simulink model "SMPMSM"  (R2018a)
settings: Solver=VariableStepAuto  StartTime=0.0  StopTime=1  MaxStep=1e-5  RelTol=1e-3
libraries: powerlib x27, simulink x5, powerlib_meascontrol x2
settings Model: Creator=Ogün Altun  LastModifiedBy=Ogün Altun
settings SolverCC: ZeroCrossAlgorithm=Adaptive
settings DebuggingCC: MaxConsecutiveZCsMsg=none

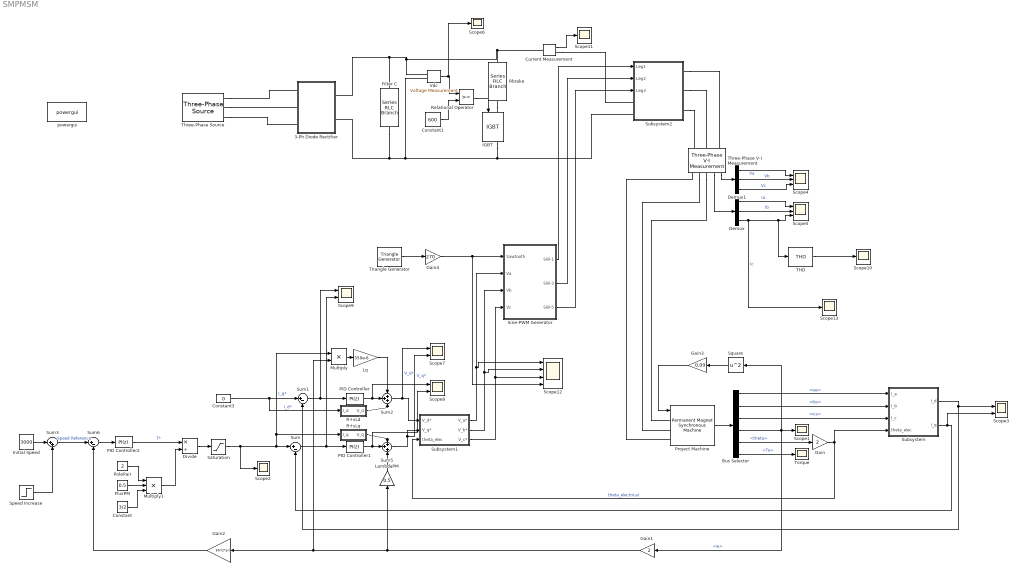
== system SMPMSM ==
  3-Ph Diode Rectifier : Subsystem
  Bus Selector : BusSelector  OutputSignals=ias,ibs,ics,w,theta,Te
  Constant : Constant  Value=3/2
  Constant1 : Constant  Value=600
  Constant3 : Constant  Value=0
  Current Measurement : powerlib/Measurements/Current Measurement  PhasorSimulation=off  OutputType=Complex  PSBequivalent=0
  Demux : Demux  Outputs=3
  Demux1 : Demux  Outputs=3
  Divide : Product  Inputs=*/
  Filter C : powerlib/Elements/Series RLC Branch  LConnTagsString=__new0  RConnTagsString=__new0  BranchType=C  Resistance=1  Inductance=1e-3  SetiL0=off  InitialCurrent=0  Capacitance=220e-6  Setx0=off  InitialVoltage=0  Measurements=None
  FluxPM : Constant  Value=0.5
  Gain : Gain  Gain=2
  Gain1 : Gain  Gain=2
  Gain2 : Gain  Gain=60/(2*pi)
  Gain3 : Gain  Gain=0.09
  Gain4 : Gain  Gain=270
  IGBT : powerlib/Power Electronics/IGBT  Ron=0.001  Lon=0  Vf=1  Tf=1e-6  Tt=2e-6  IC=0  Rs=inf  Cs=inf  Measurements=on
  "Initial Speed " : Constant  Value=3000
  LambdaPM : Gain  Gain=0.5
  Lq : Gain  Gain=350e-6
  Multiply : Product
  Multiply1 : Product  Inputs=3
  PID Controller : simulink/Continuous/PID Controller  Controller=PI  TimeDomain=Discrete-time  SampleTime=-1  IntegratorMethod=Forward Euler  FilterMethod=Forward Euler  Form=Parallel  UseFilter=on  ControllerParametersSource=internal  P=0.3  I=500  D=0  N=100  InitialConditionSource=internal  InitialConditionForIntegrator=0  InitialConditionForFilter=0  ExternalReset=none  LimitOutput=off  UpperSaturationLimit=inf  LowerSaturationLimit=-inf  LinearizeAsGain=on  AntiWindupMode=none  Kb=1  TrackingMode=off  Kt=1  PParamMin=[]  PParamMax=[]  IParamMin=[]  IParamMax=[]  DParamMin=[]  DParamMax=[]  NParamMin=[]  NParamMax=[]  KbParamMin=[]  KbParamMax=[]  KtParamMin=[]  KtParamMax=[]  POutMin=[]  POutMax=[]  IOutMin=[]  IOutMax=[]  DOutMin=[]  DOutMax=[]  NOutMin=[]  NOutMax=[]  KbOutMin=[]  KbOutMax=[]  KtOutMin=[]  KtOutMax=[]  IntegratorOutMin=[]  IntegratorOutMax=[]  FilterOutMin=[]  FilterOutMax=[]  SumOutMin=[]  SumOutMax=[]  SumI1OutMin=[]  SumI1OutMax=[]  SumI2OutMin=[]  SumI2OutMax=[]  SumI3OutMin=[]  SumI3OutMax=[]  SumDOutMin=[]  SumDOutMax=[]  SaturationOutMin=[]  SaturationOutMax=[]  IntegratorContinuousStateAttributes=''  IntegratorStateMustResolveToSignalObject=off  IntegratorRTWStateStorageClass=Auto  FilterContinuousStateAttributes=''  FilterStateMustResolveToSignalObject=off  FilterRTWStateStorageClass=Auto  DifferentiatorICPrevScaledInput=0  DifferentiatorOutMin=[]  DifferentiatorOutMax=[]  FilterDiffOutCoefMin=[]  FilterDiffOutCoefMax=[]  SumDenOutMin=[]  SumDenOutMax=[]  SumNumOutMin=[]  SumNumOutMax=[]  ReciprocalOutMin=[]  ReciprocalOutMax=[]  DivideOutMin=[]  DivideOutMax=[]  TunerSelectOption=Transfer Function Based (PID Tuner App)
  PID Controller1 : simulink/Continuous/PID Controller  Controller=PI  TimeDomain=Discrete-time  SampleTime=-1  IntegratorMethod=Forward Euler  FilterMethod=Forward Euler  Form=Parallel  UseFilter=on  ControllerParametersSource=internal  P=0.3  I=500  D=0  N=100  InitialConditionSource=internal  InitialConditionForIntegrator=0  InitialConditionForFilter=0  ExternalReset=none  LimitOutput=off  UpperSaturationLimit=inf  LowerSaturationLimit=-inf  LinearizeAsGain=on  AntiWindupMode=none  Kb=1  TrackingMode=off  Kt=1  PParamMin=[]  PParamMax=[]  IParamMin=[]  IParamMax=[]  DParamMin=[]  DParamMax=[]  NParamMin=[]  NParamMax=[]  KbParamMin=[]  KbParamMax=[]  KtParamMin=[]  KtParamMax=[]  POutMin=[]  POutMax=[]  IOutMin=[]  IOutMax=[]  DOutMin=[]  DOutMax=[]  NOutMin=[]  NOutMax=[]  KbOutMin=[]  KbOutMax=[]  KtOutMin=[]  KtOutMax=[]  IntegratorOutMin=[]  IntegratorOutMax=[]  FilterOutMin=[]  FilterOutMax=[]  SumOutMin=[]  SumOutMax=[]  SumI1OutMin=[]  SumI1OutMax=[]  SumI2OutMin=[]  SumI2OutMax=[]  SumI3OutMin=[]  SumI3OutMax=[]  SumDOutMin=[]  SumDOutMax=[]  SaturationOutMin=[]  SaturationOutMax=[]  IntegratorContinuousStateAttributes=''  IntegratorStateMustResolveToSignalObject=off  IntegratorRTWStateStorageClass=Auto  FilterContinuousStateAttributes=''  FilterStateMustResolveToSignalObject=off  FilterRTWStateStorageClass=Auto  DifferentiatorICPrevScaledInput=0  DifferentiatorOutMin=[]  DifferentiatorOutMax=[]  FilterDiffOutCoefMin=[]  FilterDiffOutCoefMax=[]  SumDenOutMin=[]  SumDenOutMax=[]  SumNumOutMin=[]  SumNumOutMax=[]  ReciprocalOutMin=[]  ReciprocalOutMax=[]  DivideOutMin=[]  DivideOutMax=[]  TunerSelectOption=Transfer Function Based (PID Tuner App)
  PID Controller2 : simulink/Continuous/PID Controller  Controller=PI  TimeDomain=Discrete-time  SampleTime=-1  IntegratorMethod=Forward Euler  FilterMethod=Forward Euler  Form=Parallel  UseFilter=on  ControllerParametersSource=internal  P=1000  I=1  D=0  N=100  InitialConditionSource=internal  InitialConditionForIntegrator=0  InitialConditionForFilter=0  ExternalReset=none  LimitOutput=off  UpperSaturationLimit=inf  LowerSaturationLimit=-inf  LinearizeAsGain=on  AntiWindupMode=none  Kb=1  TrackingMode=off  Kt=1  PParamMin=[]  PParamMax=[]  IParamMin=[]  IParamMax=[]  DParamMin=[]  DParamMax=[]  NParamMin=[]  NParamMax=[]  KbParamMin=[]  KbParamMax=[]  KtParamMin=[]  KtParamMax=[]  POutMin=[]  POutMax=[]  IOutMin=[]  IOutMax=[]  DOutMin=[]  DOutMax=[]  NOutMin=[]  NOutMax=[]  KbOutMin=[]  KbOutMax=[]  KtOutMin=[]  KtOutMax=[]  IntegratorOutMin=[]  IntegratorOutMax=[]  FilterOutMin=[]  FilterOutMax=[]  SumOutMin=[]  SumOutMax=[]  SumI1OutMin=[]  SumI1OutMax=[]  SumI2OutMin=[]  SumI2OutMax=[]  SumI3OutMin=[]  SumI3OutMax=[]  SumDOutMin=[]  SumDOutMax=[]  SaturationOutMin=[]  SaturationOutMax=[]  IntegratorContinuousStateAttributes=''  IntegratorStateMustResolveToSignalObject=off  IntegratorRTWStateStorageClass=Auto  FilterContinuousStateAttributes=''  FilterStateMustResolveToSignalObject=off  FilterRTWStateStorageClass=Auto  DifferentiatorICPrevScaledInput=0  DifferentiatorOutMin=[]  DifferentiatorOutMax=[]  FilterDiffOutCoefMin=[]  FilterDiffOutCoefMax=[]  SumDenOutMin=[]  SumDenOutMax=[]  SumNumOutMin=[]  SumNumOutMax=[]  ReciprocalOutMin=[]  ReciprocalOutMax=[]  DivideOutMin=[]  DivideOutMax=[]  TunerSelectOption=Transfer Function Based (PID Tuner App)
  PolePair : Constant  Value=2
  Project Machine : powerlib/Machines/Permanent Magnet Synchronous Machine  NbPhases=3  FluxDistribution=Sinusoidal  RotorType=Round  MechanicalLoad=Torque Tm  PresetModel=No  ShowDetailedParameters=on  MeasurementBus=on  Resistance=16e-3  Inductance=8.5e-3  dqInductances=[8.5e-3,8.5e-3]  La=350e-6  MachineConstant=Flux linkage established by magnets (V.s)  Flux=0.5  VoltageCst=181.3799  TorqueCst=1.5  Flat=120  Mechanical=[250 0 2 0]  PolePairs=4  InitialConditions=[157,0, 0,0]  InitialConditions5ph=[0 0 0 0 0 0]  TsPowergui=0  TsBlock=-1  RefAngle=Aligned with phase A axis (original Park)
      settings: SourceProductName=Simscape Power Systems
  R+sLd : Subsystem
  R+sLq : Subsystem
  Rbrake : powerlib/Elements/Series RLC Branch  LConnTagsString=__new0  RConnTagsString=__new0  BranchType=R  Resistance=10  Inductance=1e-3  SetiL0=off  InitialCurrent=0  Capacitance=1e-3  Setx0=off  InitialVoltage=0  Measurements=None
  Relational Operator : RelationalOperator  OutDataTypeStr=boolean  RndMeth=Simplest
  Saturation : Saturate  UpperLimit=1700  LowerLimit=-1700
  Scope{1..2,6,10..11,13} (6 alike) : Scope
  Scope12 : Scope  NumInputPorts=4
  Scope{3,7..9} (4 alike) : Scope  NumInputPorts=2
  Scope4 : Scope  NumInputPorts=3
  Scope5 : Scope  NumInputPorts=3
  Sine-PWM Generator : Subsystem
  Speed Increase : Step  After=300  SampleTime=0
  Square : Math  Operator=square  SaturateOnIntegerOverflow=on
  Subsystem : Subsystem
  Subsystem1 : Subsystem
  Subsystem2 : Subsystem
  Sum : Sum  Inputs=|+-
  Sum1 : Sum  Inputs=|+-
  Sum2 : Sum  Inputs=+++
  Sum3 : Sum  Inputs=|++
  Sum5 : Sum  Inputs=+++
  Sum6 : Sum  Inputs=|+-
  THD : powerlib_meascontrol/Measurements/THD  Freq=50  Ts=0
  Three-Phase V-I Measurement : powerlib/Measurements/Three-Phase V-I Measurement  VoltageMeasurement=phase-to-phase  SetLabelV=off  LabelV=Vabc  Vpu=off  VpuLL=off  CurrentMeasurement=yes  SetLabelI=off  LabelI=Iabc  Ipu=off  Pbase=100e6  Vbase=500e3  OutputType=Complex  PhasorSimulation=off  PSBequivalent=0
  Three-Phase Source : powerlib/Electrical Sources/Three-Phase Source  InternalConnection=Yg  VoltagePhases=off  Voltage=400  PhaseAngle=0  Voltage_phases=[25e3 25e3 25e3]/sqrt(3)  PhaseAngles_phases=[0 -120 +120]  Frequency=50  NonIdealSource=off  SpecifyImpedance=off  Resistance=0.8929  Inductance=16.58e-3  ShortCircuitLevel=100e6  BaseVoltage=25e3  XRratio=7  BusType=swing  Pref=10e3  Qref=0  Prefabc=[10e3, 10e3, 10e3]  Qrefabc=[0, 0, 0]  Qmin=-inf  Qmax=inf
  Torque : Scope
  Triangle Generator : powerlib_meascontrol/Pulse & Signal Generators/Triangle Generator  Freq=2475  Phase=180  Ts=0
  Vdc : powerlib/Measurements/Voltage Measurement  PhasorSimulation=off  OutputType=Complex  PSBequivalent=0
  powergui : powerlib/powergui  Priority=1  SimulationMode=Continuous  SampleTime=50e-6  frequency=60  Iterations=50  frequencyindice=0  Pbase=100e6  ErrMax=1e-4  UnitsV=kV  UnitsW=MW  buscounter=0  FunctionMessages=off  echomessages=off  EnableUseOfTLC=off  CurrentSourceSwitches=off  DisableSnubberDevices=off  DisableRonSwitches=off  DisableVfSwitches=off  DisplayEquations=off  SolverType=Tustin/Backward Euler (TBE)  Interpol=off  ExternalGateDelay=off  methode=off  Ts=100  x0status=blocks  SPID=on  SwTol=0  HookPort=off  RestoreLinks=warning  ResistiveCurrentMeasurement=off  Frange=[0:2:500]  Ylog=off  Xlog=on  ShowGrid=off  save=off  variable=ZData  structure=ic_sv  ZoomFFT=off  StartTime=0.5  cycles=20  DisplayStyle=1  fundamental=50  FreqAxis=on  MaxFrequency=50*60  frequencyindicesteady=1  RmsSteady=1  display=off
  wires:
  Bus Selector/1 -> Subsystem/1(I_a)  "<ias>"
  Bus Selector/2 -> Subsystem/2(I_b)  "<ibs>"
  Bus Selector/3 -> Subsystem/3(I_c)  "<ics>"
  Bus Selector/4 -> Square/1, Scope1/1, Gain1/1  "<w>"
  Bus Selector/5 -> Gain/1  "<theta>"
  Bus Selector/6 -> Torque/1  "<Te>"
  Gain/1 -> Subsystem/4(theta_elec), Subsystem1/3(theta_elec)  "theta_electrical"
  Sum/1 -> Scope9/2, PID Controller1/1
  Sum1/1 -> Scope9/1, PID Controller/1
  Subsystem/1(I_d) -> Sum1/2, Scope3/1
  Constant3/1 -> Sum1/1, R+sLd/1(I_d)  "I_d*"
  Divide/1 -> Saturation/1
  Subsystem/2(I_q) -> Scope3/2, Sum/2
  Subsystem1/1(V_a*) -> Scope12/1, Sine-PWM Generator/2(Va)
  Subsystem1/3(V_c*) -> Scope12/3, Sine-PWM Generator/4(Vc)
  Gain1/1 -> Multiply/2, Gain2/1, LambdaPM/1
  Sum5/1 -> Scope7/2, Subsystem1/2(V_q*)  "V_q*"
  Sum2/1 -> Scope7/1, Subsystem1/1(V_d*)  "V_d*"
  LambdaPM/1 -> Sum5/3
  Multiply/1 -> Lq/1
  Lq/1 -> Sum2/1
  PID Controller1/1 -> Scope8/2, Sum5/2
  PID Controller/1 -> Scope8/1, Sum2/2
  Gain2/1 -> Sum6/2
  Sum6/1 -> PID Controller2/1
  PID Controller2/1 -> Divide/1  "T*"
  PolePair/1 -> Multiply1/1
  FluxPM/1 -> Multiply1/2
  Constant/1 -> Multiply1/3
  Multiply1/1 -> Divide/2
  Saturation/1 -> Scope2/1, Multiply/1, R+sLq/1(I_q), Sum/1  "I_q*"
  Relational Operator/1 -> IGBT/1
  Vdc/1 -> Scope6/1, Relational Operator/1
  Constant1/1 -> Relational Operator/2
  Sine-PWM Generator/1(SW-1) -> Subsystem2/1(Leg1)
  Sine-PWM Generator/2(SW-3) -> Subsystem2/2(Leg2)
  Sine-PWM Generator/3(SW-5) -> Subsystem2/3(Leg3)
  Project Machine/1 -> Bus Selector/1
  Gain3/1 -> Project Machine/1
  Square/1 -> Gain3/1
  Three-Phase V-I Measurement/1 -> Demux1/1
  Three-Phase V-I Measurement/2 -> Demux/1
  Demux/1 -> Scope5/1  "Ia"
  Demux/2 -> Scope5/2  "Ib"
  Demux1/2 -> Scope4/2  "Vb"
  Demux1/1 -> Scope4/1  "Va"
  Demux1/3 -> Scope4/3  "Vc"
  "Initial Speed "/1 -> Sum3/1
  Sum3/1 -> Sum6/1  "Speed Reference"
  Triangle Generator/1 -> Gain4/1
  Subsystem1/2(V_b*) -> Scope12/2, Sine-PWM Generator/3(Vb)
  Gain4/1 -> Scope12/4, Sine-PWM Generator/1("Sawtooth ")
  Speed Increase/1 -> Sum3/2
  R+sLq/1(V_q) -> Sum5/1
  R+sLd/1(V_d) -> Sum2/3
  THD/1 -> Scope10/1
  Demux/3 -> Scope13/1, THD/1, Scope5/3  "Ic"
  Current Measurement/1 -> Scope11/1
  connections:
  Rbrake/RConn1 -- IGBT/LConn1
  Three-Phase Source/RConn3 -- 3-Ph Diode Rectifier/LConn3
  Three-Phase Source/RConn1 -- 3-Ph Diode Rectifier/LConn1
  Three-Phase Source/RConn2 -- 3-Ph Diode Rectifier/LConn2
  IGBT/RConn1 -- Vdc/LConn2 -- Filter C/RConn1 -- 3-Ph Diode Rectifier/RConn2 -- Subsystem2/LConn2
  Subsystem2/RConn1 -- Three-Phase V-I Measurement/LConn1
  Three-Phase V-I Measurement/RConn2 -- Project Machine/LConn2
  Three-Phase V-I Measurement/RConn3 -- Project Machine/LConn3
  Three-Phase V-I Measurement/RConn1 -- Project Machine/LConn1
  Subsystem2/RConn2 -- Three-Phase V-I Measurement/LConn2
  Subsystem2/RConn3 -- Three-Phase V-I Measurement/LConn3
  Filter C/LConn1 -- 3-Ph Diode Rectifier/RConn1 -- Rbrake/LConn1 -- Current Measurement/LConn1 -- Vdc/LConn1
  Current Measurement/RConn1 -- Subsystem2/LConn1

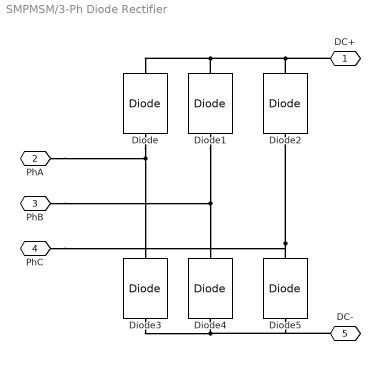
== system SMPMSM/3-Ph Diode Rectifier ==
  Diode{,1..5} (6 alike) : powerlib/Power Electronics/Diode  Ron=0.0001  Lon=0  Vf=0  IC=0  UseSnubber=0  Rs=inf  Cs=0  Measurements=off
  DC+ : PMIOPort  Side=Right
  PhA : PMIOPort  Port=2  Side=Left
  PhB : PMIOPort  Port=3  Side=Left
  PhC : PMIOPort  Port=4  Side=Left
  DC- : PMIOPort  Port=5  Side=Right
  connections:
  Diode3/LConn1 -- DC-/RConn1 -- Diode5/LConn1 -- Diode4/LConn1
  Diode2/RConn1 -- Diode1/RConn1 -- Diode/RConn1 -- DC+/RConn1
  Diode1/LConn1 -- PhB/RConn1 -- Diode4/RConn1
  Diode5/RConn1 -- Diode2/LConn1 -- PhC/RConn1
  Diode/LConn1 -- Diode3/RConn1 -- PhA/RConn1

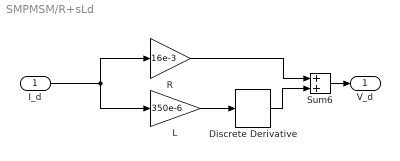
== system SMPMSM/R+sLd ==
  I_d : Inport
  Discrete Derivative : simulink/Discrete/Discrete Derivative  gainval=1.0  ICPrevScaledInput=0.0  OutMin=[]  OutMax=[]  OutDataType=fixdt(1, 16)  OutScaling=2^-10  DoSatur=off
  L : Gain  Gain=350e-6
  R : Gain  Gain=16e-3
  Sum6 : Sum
  V_d : Outport
  wires:
  I_d/1 -> R/1, L/1
  Sum6/1 -> V_d/1
  Discrete Derivative/1 -> Sum6/2
  R/1 -> Sum6/1
  L/1 -> Discrete Derivative/1

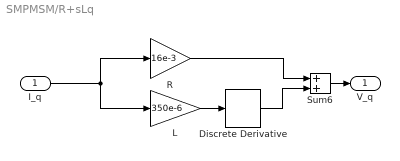
== system SMPMSM/R+sLq ==
  I_q : Inport
  Discrete Derivative : simulink/Discrete/Discrete Derivative  gainval=1.0  ICPrevScaledInput=0.0  InputProcessing=Inherited  OutMin=[]  OutMax=[]  OutDataType=fixdt(1, 16)  OutScaling=2^-10  DoSatur=off
  L : Gain  Gain=350e-6
  R : Gain  Gain=16e-3
  Sum6 : Sum
  V_q : Outport
  wires:
  L/1 -> Discrete Derivative/1
  R/1 -> Sum6/1
  Discrete Derivative/1 -> Sum6/2
  Sum6/1 -> V_q/1
  I_q/1 -> L/1, R/1

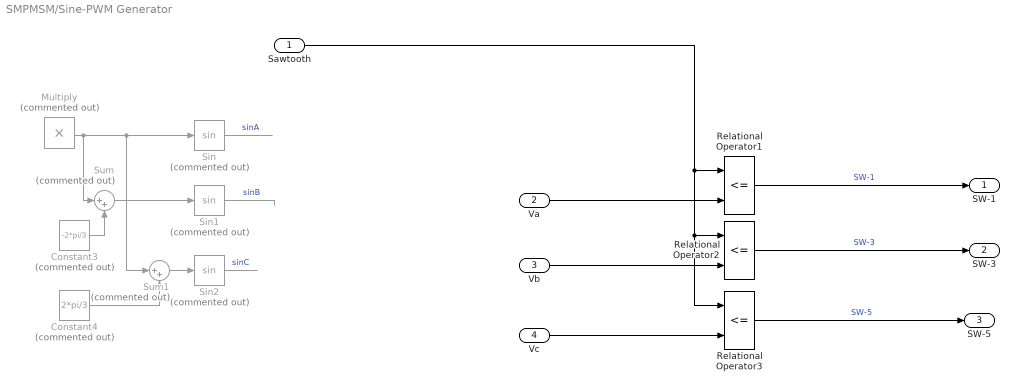
== system SMPMSM/Sine-PWM Generator ==
  "Sawtooth " : Inport
  Va : Inport  Port=2
  Vb : Inport  Port=3
  Vc : Inport  Port=4
  Constant3 : Constant  Commented=on  Value=-2*pi/3
  Constant4 : Constant  Commented=on  Value=2*pi/3
  Multiply : Product  Commented=on
  Relational Operator1 : RelationalOperator  Operator=<=  OutDataTypeStr=boolean  RndMeth=Simplest
  Relational Operator2 : RelationalOperator  Operator=<=  OutDataTypeStr=boolean  RndMeth=Simplest
  Relational Operator3 : RelationalOperator  Operator=<=  OutDataTypeStr=boolean  RndMeth=Simplest
  Sin : Trigonometry  Commented=on
  Sin1 : Trigonometry  Commented=on
  Sin2 : Trigonometry  Commented=on
  Sum : Sum  Commented=on  Inputs=|++
  Sum1 : Sum  Commented=on  Inputs=|++
  SW-1 : Outport
  SW-3 : Outport  Port=2
  SW-5 : Outport  Port=3
  wires:
  Sin/1 -> ?  "sinA"
  "Sawtooth "/1 -> Relational Operator3/1, Relational Operator2/1, Relational Operator1/1
  Constant3/1 -> Sum/2
  Constant4/1 -> Sum1/2
  Sum/1 -> Sin1/1
  Sum1/1 -> Sin2/1
  Sin2/1 -> ?  "sinC"
  Multiply/1 -> Sum/1, Sum1/1, Sin/1
  Sin1/1 -> ?  "sinB"
  Relational Operator2/1 -> SW-3/1  "SW-3"
  Relational Operator1/1 -> SW-1/1  "SW-1"
  Relational Operator3/1 -> SW-5/1  "SW-5"
  Vc/1 -> Relational Operator3/2
  Va/1 -> Relational Operator1/2
  Vb/1 -> Relational Operator2/2

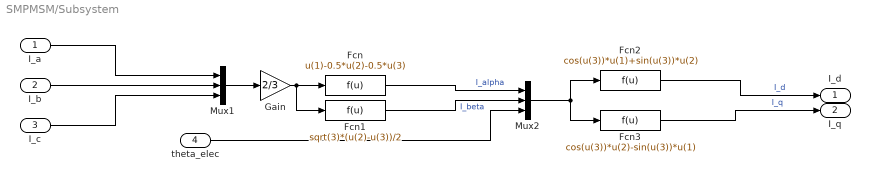
== system SMPMSM/Subsystem ==
  I_a : Inport
  I_b : Inport  Port=2
  I_c : Inport  Port=3
  theta_elec : Inport  Port=4
  Fcn : Fcn  Expr=u(1)-0.5*u(2)-0.5*u(3)
  Fcn1 : Fcn  Expr=sqrt(3)*(u(2)-u(3))/2
  Fcn2 : Fcn  Expr=cos(u(3))*u(1)+sin(u(3))*u(2)
  Fcn3 : Fcn  Expr=cos(u(3))*u(2)-sin(u(3))*u(1)
  Gain : Gain  Gain=2/3
  Mux1 : Mux  Inputs=3
  Mux2 : Mux  Inputs=3
  I_d : Outport
  I_q : Outport  Port=2
  wires:
  theta_elec/1 -> Mux2/3
  Fcn1/1 -> Mux2/2  "I_beta"
  Mux1/1 -> Gain/1
  Fcn/1 -> Mux2/1  "I_alpha"
  Mux2/1 -> Fcn3/1, Fcn2/1
  Fcn3/1 -> I_q/1  "I_q"
  I_b/1 -> Mux1/2
  I_a/1 -> Mux1/1
  Fcn2/1 -> I_d/1  "I_d"
  I_c/1 -> Mux1/3
  Gain/1 -> Fcn1/1, Fcn/1

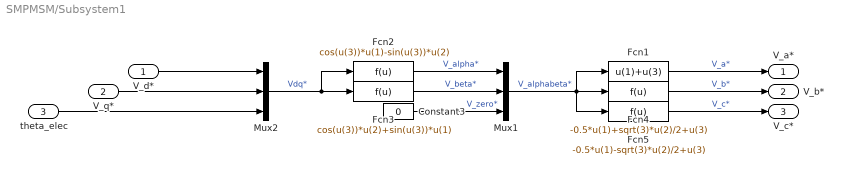
== system SMPMSM/Subsystem1 ==
  V_d* : Inport
  V_q* : Inport  Port=2
  theta_elec : Inport  Port=3
  Constant3 : Constant  Value=0
  Fcn1 : Fcn  Expr=u(1)+u(3)
  Fcn2 : Fcn  Expr=cos(u(3))*u(1)-sin(u(3))*u(2)
  Fcn3 : Fcn  Expr=cos(u(3))*u(2)+sin(u(3))*u(1)
  Fcn4 : Fcn  Expr=-0.5*u(1)+sqrt(3)*u(2)/2+u(3)
  Fcn5 : Fcn  Expr=-0.5*u(1)-sqrt(3)*u(2)/2+u(3)
  Mux1 : Mux  Inputs=3
  Mux2 : Mux  Inputs=3
  V_a* : Outport
  V_b* : Outport  Port=2
  V_c* : Outport  Port=3
  wires:
  Fcn5/1 -> V_c*/1  "V_c*"
  Mux2/1 -> Fcn2/1, Fcn3/1  "Vdq*"
  Fcn1/1 -> V_a*/1  "V_a*"
  Mux1/1 -> Fcn1/1, Fcn5/1, Fcn4/1  "V_alphabeta*"
  Fcn3/1 -> Mux1/2  "V_beta*"
  V_d*/1 -> Mux2/1
  Fcn2/1 -> Mux1/1  "V_alpha*"
  Fcn4/1 -> V_b*/1  "V_b*"
  Constant3/1 -> Mux1/3  "V_zero*"
  theta_elec/1 -> Mux2/3
  V_q*/1 -> Mux2/2

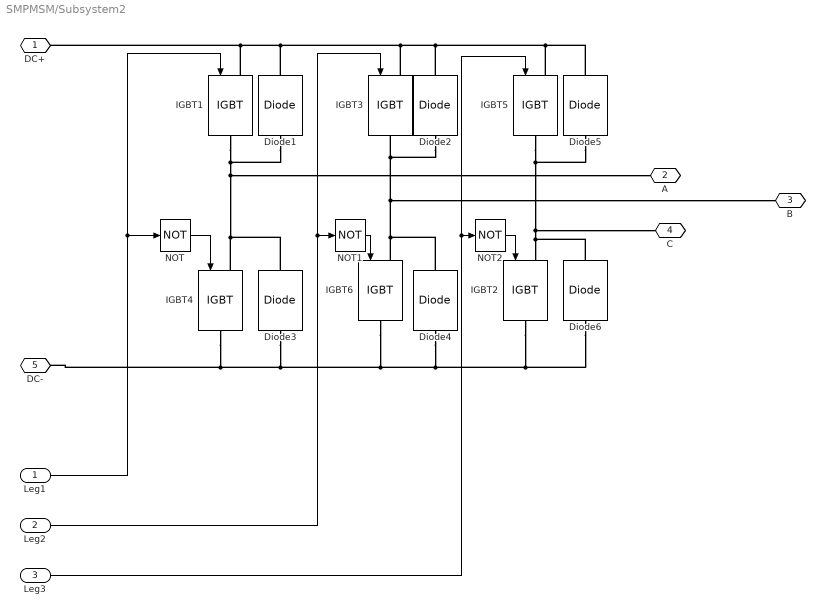
== system SMPMSM/Subsystem2 ==
  Leg1 : Inport
  Leg2 : Inport  Port=2
  Leg3 : Inport  Port=3
  Diode{1..6} (6 alike) : powerlib/Power Electronics/Diode  Ron=0.0001  Lon=0  Vf=0  IC=0  UseSnubber=0  Rs=inf  Cs=0  Measurements=off
  IGBT{1..6} (6 alike) : powerlib/Power Electronics/IGBT  Ron=0.001  Lon=0  Vf=0  Tf=1e-6  Tt=2e-6  IC=0  Rs=inf  Cs=inf  Measurements=off
  NOT : Logic  Operator=NOT  IconShape=distinctive  AllPortsSameDT=off  OutDataTypeStr=boolean
  NOT1 : Logic  Operator=NOT  IconShape=distinctive  AllPortsSameDT=off  OutDataTypeStr=boolean
  NOT2 : Logic  Operator=NOT  IconShape=distinctive  AllPortsSameDT=off  OutDataTypeStr=boolean
  DC+ : PMIOPort  Side=Left
  A : PMIOPort  Port=2  Side=Right
  B : PMIOPort  Port=3  Side=Right
  C : PMIOPort  Port=4  Side=Right
  DC- : PMIOPort  Port=5  Side=Left
  wires:
  NOT1/1 -> IGBT6/1
  Leg3/1 -> IGBT5/1, NOT2/1
  Leg2/1 -> NOT1/1, IGBT3/1
  Leg1/1 -> NOT/1, IGBT1/1
  NOT/1 -> IGBT4/1
  NOT2/1 -> IGBT2/1
  connections:
  IGBT5/RConn1 -- Diode5/LConn1 -- IGBT2/LConn1 -- Diode6/RConn1 -- C/RConn1
  IGBT4/LConn1 -- Diode3/RConn1 -- IGBT1/RConn1 -- Diode1/LConn1 -- A/RConn1
  Diode5/RConn1 -- IGBT5/LConn1 -- Diode2/RConn1 -- IGBT3/LConn1 -- Diode1/RConn1 -- DC+/RConn1 -- IGBT1/LConn1
  IGBT3/RConn1 -- IGBT6/LConn1 -- Diode4/RConn1 -- B/RConn1 -- Diode2/LConn1
  IGBT6/RConn1 -- Diode6/LConn1 -- IGBT2/RConn1 -- Diode4/LConn1 -- IGBT4/RConn1 -- DC-/RConn1 -- Diode3/LConn1
